simulink model "FL_s_inv_int"  (R2023b)
settings: Solver=VariableStepAuto  StartTime=0.0  StopTime=20  RelTol=1e-7
values from neighbouring files (symbols this model uses):
  ki = input(5)    [FL_s_inv_control_law_int.m]    (also in FL_s_v_control_law_int.m = input(7))
undefined symbols (not defined in the file or in its folder): Disturbo
settings Model: Creator=giov_russo  LastModifiedBy=miche
settings SolverCC: AlgebraicLoopSolver=TrustRegion
settings DebuggingCC: UnconnectedInputMsg=warning  UnconnectedOutputMsg=warning  UnconnectedLineMsg=warning
settings ModelReferenceCC: EnableRefExpFcnMdlSchedulingChecks=on

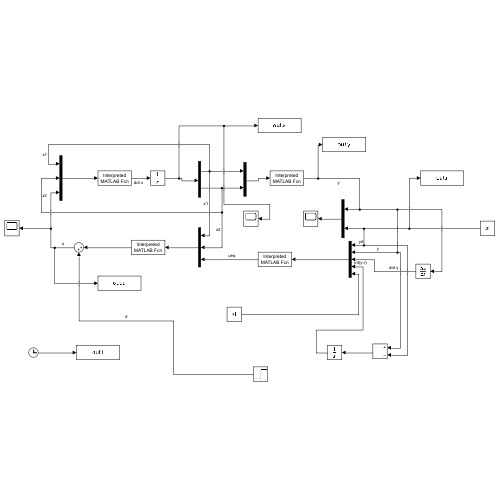
[thumbnail: Simulink's stored preview of the top-level diagram]
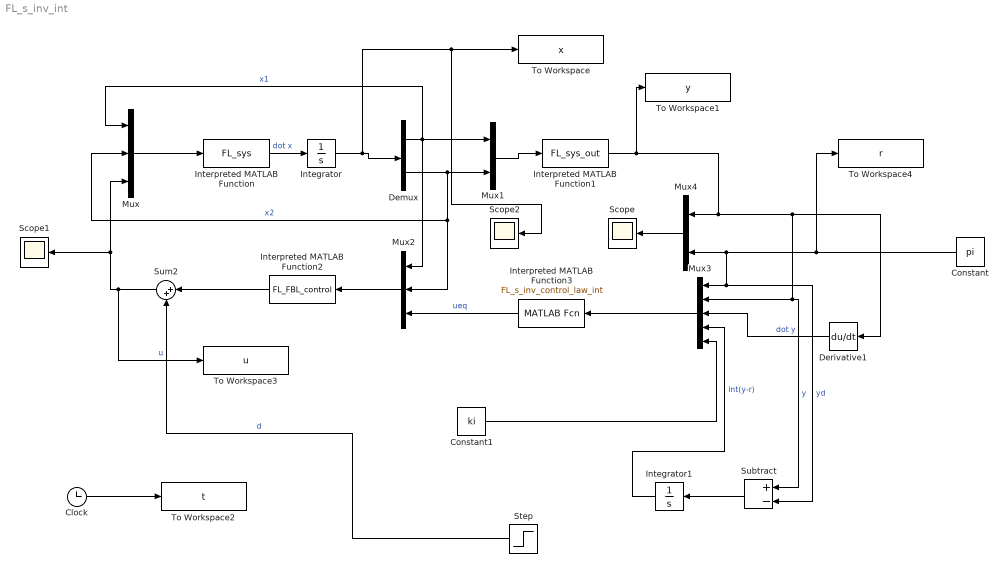
== system FL_s_inv_int ==
  Clock : Clock
  Constant : Constant  Value=pi
  Constant1 : Constant  Value=ki
  Demux : Demux  Outputs=2
  Derivative1 : Derivative
  Integrator : Integrator
  Integrator1 : Integrator
  Interpreted MATLAB Function : MATLABFcn  MATLABFcn=FL_sys  OutputDimensions=2
  Interpreted MATLAB Function1 : MATLABFcn  MATLABFcn=FL_sys_out  OutputDimensions=1
  Interpreted MATLAB Function2 : MATLABFcn  MATLABFcn=FL_FBL_control  OutputDimensions=1
  Interpreted MATLAB Function3 : MATLABFcn  MATLABFcn=FL_s_inv_control_law_int  OutputDimensions=1
  Mux : Mux  Inputs=3
  Mux1 : Mux  Inputs=2
  Mux2 : Mux  Inputs=3
  Mux3 : Mux  Inputs=5
  Mux4 : Mux  Inputs=2
  Scope : Scope
  Scope1 : Scope
  Scope2 : Scope
  Step : Step  Time=5  After=Disturbo  SampleTime=0
  Subtract : Sum  Inputs=+-
  Sum2 : Sum  Inputs=|++
  To Workspace : ToWorkspace  VariableName=x  SampleTime=-1
  To Workspace1 : ToWorkspace  VariableName=y  SampleTime=-1
  To Workspace2 : ToWorkspace  VariableName=t  SampleTime=-1
  To Workspace3 : ToWorkspace  VariableName=u  SampleTime=-1
  To Workspace4 : ToWorkspace  VariableName=r  SampleTime=-1
  wires:
  Mux/1 -> Interpreted MATLAB Function/1
  Interpreted MATLAB Function/1 -> Integrator/1  "dot x"
  Integrator/1 -> Scope2/1, To Workspace/1, Demux/1
  Demux/2 -> Mux/2, Mux2/2, Mux1/2  "x2"
  Mux1/1 -> Interpreted MATLAB Function1/1
  Mux2/1 -> Interpreted MATLAB Function2/1
  Mux3/1 -> Interpreted MATLAB Function3/1
  Mux4/1 -> Scope/1
  Demux/1 -> Mux/1, Mux1/1, Mux2/1  "x1"
  Interpreted MATLAB Function3/1 -> Mux2/3  "ueq"
  Interpreted MATLAB Function1/1 -> To Workspace1/1, Derivative1/1, Subtract/1, Mux3/2, Mux4/1  "y"
  Clock/1 -> To Workspace2/1
  Constant/1 -> To Workspace4/1, Subtract/2, Mux3/1, Mux4/2  "yd"
  Derivative1/1 -> Mux3/3  "dot y"
  Subtract/1 -> Integrator1/1
  Integrator1/1 -> Mux3/4  "int(y-r)"
  Step/1 -> Sum2/2  "d"
  Interpreted MATLAB Function2/1 -> Sum2/1
  Sum2/1 -> To Workspace3/1, Scope1/1, Mux/3  "u"
  Constant1/1 -> Mux3/5
